simulink model "Autopilot_q_running1"  (R2021a)
settings: Solver=ode4  StartTime=0.0  StopTime=168  FixedStep=0.01  RelTol=1e-3
undefined symbols (not defined in the file or in its folder): Aero_cofficients, Earth, Plane_state_store, Structural_data, Thrust_data_store, WGS84
libraries: pid_lib x12, aerolibactuator x5, aerolibfltsims x2, aerolibanim x1, simulink x1, aerolibtransform2 x1, shared6dof x1, sim3dlib x1, uavsim3dlib x1
(part 2 of 3)

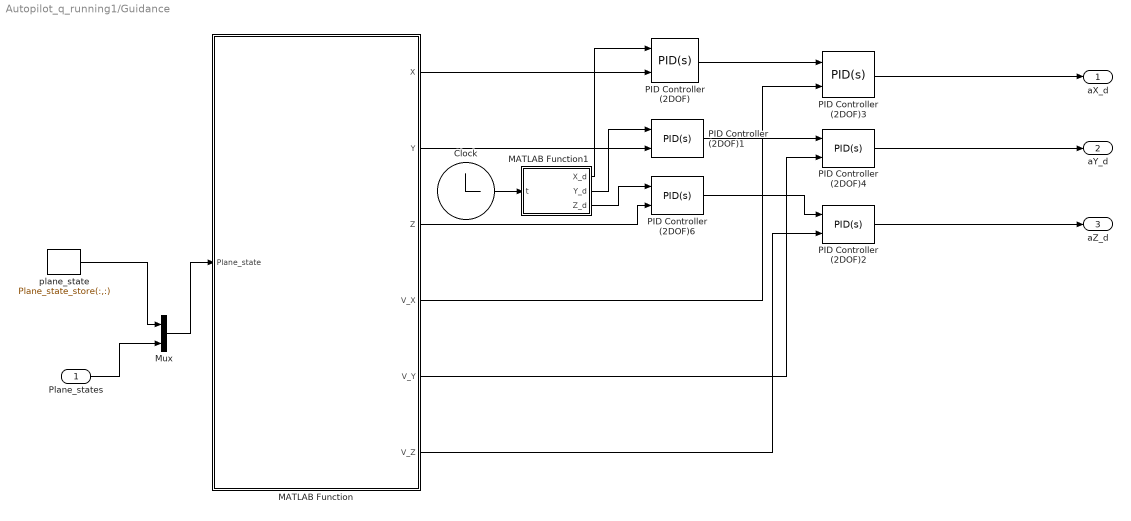
== system Autopilot_q_running1/Guidance ==
  Plane_states : Inport
  Clock : Clock
      settings: Decimation=200
  MATLAB Function : MATLAB Function  TreatAsAtomicUnit=on
  MATLAB Function1 : MATLAB Function  TreatAsAtomicUnit=on
  Mux : Mux  Inputs=2
  PID Controller (2DOF) : pid_lib/PID Controller (2DOF)  Controller=PID  Form=Parallel  TimeDomain=Continuous-time  UseExternalTs=off  SampleTime=-1  IntegratorMethod=Forward Euler  FilterMethod=Forward Euler  ControllerParametersSource=internal  P=0.4  I=0  D=0  UseFilter=on  N=100  b=1  c=1  TunerSelectOption=Transfer Function Based (PID Tuner App)  InitialConditionSource=internal  InitialConditionForIntegrator=0  InitialConditionForFilter=0  DifferentiatorICPrevScaledInput=0  ExternalReset=none  TrackingMode=off  Kt=1  LimitOutput=off  SatLimitsSource=internal  UpperSaturationLimit=inf  LowerSaturationLimit=-inf  LinearizeAsGain=on  AntiWindupMode=none  Kb=1  POutMin=[]  POutMax=[]  IOutMin=[]  IOutMax=[]  DOutMin=[]  DOutMax=[]  NOutMin=[]  NOutMax=[]  bOutMin=[]  bOutMax=[]  cOutMin=[]  cOutMax=[]  SumOutMin=[]  SumOutMax=[]  SaturationOutMin=[]  SaturationOutMax=[]  PParamMin=[]  PParamMax=[]  IParamMin=[]  IParamMax=[]  DParamMin=[]  DParamMax=[]  NParamMin=[]  NParamMax=[]  bParamMin=[]  bParamMax=[]  cParamMin=[]  cParamMax=[]  KbParamMin=[]  KbParamMax=[]  KtParamMin=[]  KtParamMax=[]  KbOutMin=[]  KbOutMax=[]  KtOutMin=[]  KtOutMax=[]  IntegratorOutMin=[]  IntegratorOutMax=[]  FilterOutMin=[]  FilterOutMax=[]  SumI1OutMin=[]  SumI1OutMax=[]  SumI2OutMin=[]  SumI2OutMax=[]  SumI3OutMin=[]  SumI3OutMax=[]  SumI4OutMin=[]  SumI4OutMax=[]  SumDOutMin=[]  SumDOutMax=[]  Sum1OutMin=[]  Sum1OutMax=[]  Sum2OutMin=[]  Sum2OutMax=[]  Sum3OutMin=[]  Sum3OutMax=[]  DifferentiatorOutMin=[]  DifferentiatorOutMax=[]  FilterDiffOutCoefMin=[]  FilterDiffOutCoefMax=[]  ReciprocalOutMin=[]  ReciprocalOutMax=[]  SumDenOutMin=[]  SumDenOutMax=[]  SumNumOutMin=[]  SumNumOutMax=[]  DivideOutMin=[]  DivideOutMax=[]  UdiffTsProdOutMin=[]  UdiffTsProdOutMax=[]  NTsProdOutMin=[]  NTsProdOutMax=[]  UintegralTsProdOutMin=[]  UintegralTsProdOutMax=[]  UngainTsProdOutMin=[]  UngainTsProdOutMax=[]  IntegratorContinuousStateAttributes=''  IntegratorStateMustResolveToSignalObject=off  IntegratorRTWStateStorageClass=Auto  FilterContinuousStateAttributes=''  FilterStateMustResolveToSignalObject=off  FilterRTWStateStorageClass=Auto  ParallelPVariant=InternalParameters  IdealPVariant=Disabled  IVariant=InternalParameters  DVariant=InternalParameters  bVariant=InternalParameters  cVariant=InternalParameters  IntegratorVariant=Continuous  SatVariant=Disabled  AWVariant=Passthrough  PCopyVariant=Disabled  TRVariant=Disabled  FdbkBlocksVariant=Forward  IdealPFdbkVariant=Disabled  SatFdbkVariant=Disabled  DerivativeFilterVariant=ContFilter  NVariant=InternalParameters  NCopyVariant=Disabled  FilterICVariant=InternalICsFilter  IntegratorICVariant=InternalICs  ExternalResetVariant=Disabled  TRSumVariant=Passthrough  SumFdbkVariant=Disabled  SumVariant=Sum_PID  TsampFilterVariant=InternalTs  TsampNgainVariant=Passthrough  TsampIntegralVariant=Passthrough  ExternalSaturationOutDataTypeStr=Inherit: Same as second input
      settings: SourceProductBaseCode=SL
  PID Controller (2DOF)1 : pid_lib/PID Controller (2DOF)  Controller=PID  Form=Parallel  TimeDomain=Continuous-time  UseExternalTs=off  SampleTime=-1  IntegratorMethod=Forward Euler  FilterMethod=Forward Euler  ControllerParametersSource=internal  P=0.4  I=0  D=0  UseFilter=on  N=100  b=1  c=1  TunerSelectOption=Transfer Function Based (PID Tuner App)  InitialConditionSource=internal  InitialConditionForIntegrator=0  InitialConditionForFilter=0  DifferentiatorICPrevScaledInput=0  ExternalReset=none  TrackingMode=off  Kt=1  LimitOutput=off  SatLimitsSource=internal  UpperSaturationLimit=inf  LowerSaturationLimit=-inf  LinearizeAsGain=on  AntiWindupMode=none  Kb=1  POutMin=[]  POutMax=[]  IOutMin=[]  IOutMax=[]  DOutMin=[]  DOutMax=[]  NOutMin=[]  NOutMax=[]  bOutMin=[]  bOutMax=[]  cOutMin=[]  cOutMax=[]  SumOutMin=[]  SumOutMax=[]  SaturationOutMin=[]  SaturationOutMax=[]  PParamMin=[]  PParamMax=[]  IParamMin=[]  IParamMax=[]  DParamMin=[]  DParamMax=[]  NParamMin=[]  NParamMax=[]  bParamMin=[]  bParamMax=[]  cParamMin=[]  cParamMax=[]  KbParamMin=[]  KbParamMax=[]  KtParamMin=[]  KtParamMax=[]  KbOutMin=[]  KbOutMax=[]  KtOutMin=[]  KtOutMax=[]  IntegratorOutMin=[]  IntegratorOutMax=[]  FilterOutMin=[]  FilterOutMax=[]  SumI1OutMin=[]  SumI1OutMax=[]  SumI2OutMin=[]  SumI2OutMax=[]  SumI3OutMin=[]  SumI3OutMax=[]  SumI4OutMin=[]  SumI4OutMax=[]  SumDOutMin=[]  SumDOutMax=[]  Sum1OutMin=[]  Sum1OutMax=[]  Sum2OutMin=[]  Sum2OutMax=[]  Sum3OutMin=[]  Sum3OutMax=[]  DifferentiatorOutMin=[]  DifferentiatorOutMax=[]  FilterDiffOutCoefMin=[]  FilterDiffOutCoefMax=[]  ReciprocalOutMin=[]  ReciprocalOutMax=[]  SumDenOutMin=[]  SumDenOutMax=[]  SumNumOutMin=[]  SumNumOutMax=[]  DivideOutMin=[]  DivideOutMax=[]  UdiffTsProdOutMin=[]  UdiffTsProdOutMax=[]  NTsProdOutMin=[]  NTsProdOutMax=[]  UintegralTsProdOutMin=[]  UintegralTsProdOutMax=[]  UngainTsProdOutMin=[]  UngainTsProdOutMax=[]  IntegratorContinuousStateAttributes=''  IntegratorStateMustResolveToSignalObject=off  IntegratorRTWStateStorageClass=Auto  FilterContinuousStateAttributes=''  FilterStateMustResolveToSignalObject=off  FilterRTWStateStorageClass=Auto  ParallelPVariant=InternalParameters  IdealPVariant=Disabled  IVariant=InternalParameters  DVariant=InternalParameters  bVariant=InternalParameters  cVariant=InternalParameters  IntegratorVariant=Continuous  SatVariant=Disabled  AWVariant=Passthrough  PCopyVariant=Disabled  TRVariant=Disabled  FdbkBlocksVariant=Forward  IdealPFdbkVariant=Disabled  SatFdbkVariant=Disabled  DerivativeFilterVariant=ContFilter  NVariant=InternalParameters  NCopyVariant=Disabled  FilterICVariant=InternalICsFilter  IntegratorICVariant=InternalICs  ExternalResetVariant=Disabled  TRSumVariant=Passthrough  SumFdbkVariant=Disabled  SumVariant=Sum_PID  TsampFilterVariant=InternalTs  TsampNgainVariant=Passthrough  TsampIntegralVariant=Passthrough  ExternalSaturationOutDataTypeStr=Inherit: Same as second input
      settings: SourceProductBaseCode=SL
  PID Controller (2DOF)2 : pid_lib/PID Controller (2DOF)  Controller=PID  Form=Parallel  TimeDomain=Continuous-time  UseExternalTs=off  SampleTime=-1  IntegratorMethod=Forward Euler  FilterMethod=Forward Euler  ControllerParametersSource=internal  P=1  I=0.0  D=0  UseFilter=on  N=100  b=1  c=1  TunerSelectOption=Transfer Function Based (PID Tuner App)  InitialConditionSource=internal  InitialConditionForIntegrator=0  InitialConditionForFilter=0  DifferentiatorICPrevScaledInput=0  ExternalReset=none  TrackingMode=off  Kt=1  LimitOutput=off  SatLimitsSource=internal  UpperSaturationLimit=inf  LowerSaturationLimit=-inf  LinearizeAsGain=on  AntiWindupMode=none  Kb=1  POutMin=[]  POutMax=[]  IOutMin=[]  IOutMax=[]  DOutMin=[]  DOutMax=[]  NOutMin=[]  NOutMax=[]  bOutMin=[]  bOutMax=[]  cOutMin=[]  cOutMax=[]  SumOutMin=[]  SumOutMax=[]  SaturationOutMin=[]  SaturationOutMax=[]  PParamMin=[]  PParamMax=[]  IParamMin=[]  IParamMax=[]  DParamMin=[]  DParamMax=[]  NParamMin=[]  NParamMax=[]  bParamMin=[]  bParamMax=[]  cParamMin=[]  cParamMax=[]  KbParamMin=[]  KbParamMax=[]  KtParamMin=[]  KtParamMax=[]  KbOutMin=[]  KbOutMax=[]  KtOutMin=[]  KtOutMax=[]  IntegratorOutMin=[]  IntegratorOutMax=[]  FilterOutMin=[]  FilterOutMax=[]  SumI1OutMin=[]  SumI1OutMax=[]  SumI2OutMin=[]  SumI2OutMax=[]  SumI3OutMin=[]  SumI3OutMax=[]  SumI4OutMin=[]  SumI4OutMax=[]  SumDOutMin=[]  SumDOutMax=[]  Sum1OutMin=[]  Sum1OutMax=[]  Sum2OutMin=[]  Sum2OutMax=[]  Sum3OutMin=[]  Sum3OutMax=[]  DifferentiatorOutMin=[]  DifferentiatorOutMax=[]  FilterDiffOutCoefMin=[]  FilterDiffOutCoefMax=[]  ReciprocalOutMin=[]  ReciprocalOutMax=[]  SumDenOutMin=[]  SumDenOutMax=[]  SumNumOutMin=[]  SumNumOutMax=[]  DivideOutMin=[]  DivideOutMax=[]  UdiffTsProdOutMin=[]  UdiffTsProdOutMax=[]  NTsProdOutMin=[]  NTsProdOutMax=[]  UintegralTsProdOutMin=[]  UintegralTsProdOutMax=[]  UngainTsProdOutMin=[]  UngainTsProdOutMax=[]  IntegratorContinuousStateAttributes=''  IntegratorStateMustResolveToSignalObject=off  IntegratorRTWStateStorageClass=Auto  FilterContinuousStateAttributes=''  FilterStateMustResolveToSignalObject=off  FilterRTWStateStorageClass=Auto  ParallelPVariant=InternalParameters  IdealPVariant=Disabled  IVariant=InternalParameters  DVariant=InternalParameters  bVariant=InternalParameters  cVariant=InternalParameters  IntegratorVariant=Continuous  SatVariant=Disabled  AWVariant=Passthrough  PCopyVariant=Disabled  TRVariant=Disabled  FdbkBlocksVariant=Forward  IdealPFdbkVariant=Disabled  SatFdbkVariant=Disabled  DerivativeFilterVariant=ContFilter  NVariant=InternalParameters  NCopyVariant=Disabled  FilterICVariant=InternalICsFilter  IntegratorICVariant=InternalICs  ExternalResetVariant=Disabled  TRSumVariant=Passthrough  SumFdbkVariant=Disabled  SumVariant=Sum_PID  TsampFilterVariant=InternalTs  TsampNgainVariant=Passthrough  TsampIntegralVariant=Passthrough  ExternalSaturationOutDataTypeStr=Inherit: Same as second input
      settings: SourceProductBaseCode=SL
  PID Controller (2DOF)3 : pid_lib/PID Controller (2DOF)  Controller=PID  Form=Parallel  TimeDomain=Continuous-time  UseExternalTs=off  SampleTime=-1  IntegratorMethod=Forward Euler  FilterMethod=Forward Euler  ControllerParametersSource=internal  P=1  I=0.0  D=0  UseFilter=on  N=100  b=1  c=1  TunerSelectOption=Transfer Function Based (PID Tuner App)  InitialConditionSource=internal  InitialConditionForIntegrator=0  InitialConditionForFilter=0  DifferentiatorICPrevScaledInput=0  ExternalReset=none  TrackingMode=off  Kt=1  LimitOutput=off  SatLimitsSource=internal  UpperSaturationLimit=inf  LowerSaturationLimit=-inf  LinearizeAsGain=on  AntiWindupMode=none  Kb=1  POutMin=[]  POutMax=[]  IOutMin=[]  IOutMax=[]  DOutMin=[]  DOutMax=[]  NOutMin=[]  NOutMax=[]  bOutMin=[]  bOutMax=[]  cOutMin=[]  cOutMax=[]  SumOutMin=[]  SumOutMax=[]  SaturationOutMin=[]  SaturationOutMax=[]  PParamMin=[]  PParamMax=[]  IParamMin=[]  IParamMax=[]  DParamMin=[]  DParamMax=[]  NParamMin=[]  NParamMax=[]  bParamMin=[]  bParamMax=[]  cParamMin=[]  cParamMax=[]  KbParamMin=[]  KbParamMax=[]  KtParamMin=[]  KtParamMax=[]  KbOutMin=[]  KbOutMax=[]  KtOutMin=[]  KtOutMax=[]  IntegratorOutMin=[]  IntegratorOutMax=[]  FilterOutMin=[]  FilterOutMax=[]  SumI1OutMin=[]  SumI1OutMax=[]  SumI2OutMin=[]  SumI2OutMax=[]  SumI3OutMin=[]  SumI3OutMax=[]  SumI4OutMin=[]  SumI4OutMax=[]  SumDOutMin=[]  SumDOutMax=[]  Sum1OutMin=[]  Sum1OutMax=[]  Sum2OutMin=[]  Sum2OutMax=[]  Sum3OutMin=[]  Sum3OutMax=[]  DifferentiatorOutMin=[]  DifferentiatorOutMax=[]  FilterDiffOutCoefMin=[]  FilterDiffOutCoefMax=[]  ReciprocalOutMin=[]  ReciprocalOutMax=[]  SumDenOutMin=[]  SumDenOutMax=[]  SumNumOutMin=[]  SumNumOutMax=[]  DivideOutMin=[]  DivideOutMax=[]  UdiffTsProdOutMin=[]  UdiffTsProdOutMax=[]  NTsProdOutMin=[]  NTsProdOutMax=[]  UintegralTsProdOutMin=[]  UintegralTsProdOutMax=[]  UngainTsProdOutMin=[]  UngainTsProdOutMax=[]  IntegratorContinuousStateAttributes=''  IntegratorStateMustResolveToSignalObject=off  IntegratorRTWStateStorageClass=Auto  FilterContinuousStateAttributes=''  FilterStateMustResolveToSignalObject=off  FilterRTWStateStorageClass=Auto  ParallelPVariant=InternalParameters  IdealPVariant=Disabled  IVariant=InternalParameters  DVariant=InternalParameters  bVariant=InternalParameters  cVariant=InternalParameters  IntegratorVariant=Continuous  SatVariant=Disabled  AWVariant=Passthrough  PCopyVariant=Disabled  TRVariant=Disabled  FdbkBlocksVariant=Forward  IdealPFdbkVariant=Disabled  SatFdbkVariant=Disabled  DerivativeFilterVariant=ContFilter  NVariant=InternalParameters  NCopyVariant=Disabled  FilterICVariant=InternalICsFilter  IntegratorICVariant=InternalICs  ExternalResetVariant=Disabled  TRSumVariant=Passthrough  SumFdbkVariant=Disabled  SumVariant=Sum_PID  TsampFilterVariant=InternalTs  TsampNgainVariant=Passthrough  TsampIntegralVariant=Passthrough  ExternalSaturationOutDataTypeStr=Inherit: Same as second input
      settings: SourceProductBaseCode=SL
  PID Controller (2DOF)4 : pid_lib/PID Controller (2DOF)  Controller=PID  Form=Parallel  TimeDomain=Continuous-time  UseExternalTs=off  SampleTime=-1  IntegratorMethod=Forward Euler  FilterMethod=Forward Euler  ControllerParametersSource=internal  P=1  I=0  D=0  UseFilter=on  N=100  b=1  c=1  TunerSelectOption=Transfer Function Based (PID Tuner App)  InitialConditionSource=internal  InitialConditionForIntegrator=0  InitialConditionForFilter=0  DifferentiatorICPrevScaledInput=0  ExternalReset=none  TrackingMode=off  Kt=1  LimitOutput=off  SatLimitsSource=internal  UpperSaturationLimit=inf  LowerSaturationLimit=-inf  LinearizeAsGain=on  AntiWindupMode=none  Kb=1  POutMin=[]  POutMax=[]  IOutMin=[]  IOutMax=[]  DOutMin=[]  DOutMax=[]  NOutMin=[]  NOutMax=[]  bOutMin=[]  bOutMax=[]  cOutMin=[]  cOutMax=[]  SumOutMin=[]  SumOutMax=[]  SaturationOutMin=[]  SaturationOutMax=[]  PParamMin=[]  PParamMax=[]  IParamMin=[]  IParamMax=[]  DParamMin=[]  DParamMax=[]  NParamMin=[]  NParamMax=[]  bParamMin=[]  bParamMax=[]  cParamMin=[]  cParamMax=[]  KbParamMin=[]  KbParamMax=[]  KtParamMin=[]  KtParamMax=[]  KbOutMin=[]  KbOutMax=[]  KtOutMin=[]  KtOutMax=[]  IntegratorOutMin=[]  IntegratorOutMax=[]  FilterOutMin=[]  FilterOutMax=[]  SumI1OutMin=[]  SumI1OutMax=[]  SumI2OutMin=[]  SumI2OutMax=[]  SumI3OutMin=[]  SumI3OutMax=[]  SumI4OutMin=[]  SumI4OutMax=[]  SumDOutMin=[]  SumDOutMax=[]  Sum1OutMin=[]  Sum1OutMax=[]  Sum2OutMin=[]  Sum2OutMax=[]  Sum3OutMin=[]  Sum3OutMax=[]  DifferentiatorOutMin=[]  DifferentiatorOutMax=[]  FilterDiffOutCoefMin=[]  FilterDiffOutCoefMax=[]  ReciprocalOutMin=[]  ReciprocalOutMax=[]  SumDenOutMin=[]  SumDenOutMax=[]  SumNumOutMin=[]  SumNumOutMax=[]  DivideOutMin=[]  DivideOutMax=[]  UdiffTsProdOutMin=[]  UdiffTsProdOutMax=[]  NTsProdOutMin=[]  NTsProdOutMax=[]  UintegralTsProdOutMin=[]  UintegralTsProdOutMax=[]  UngainTsProdOutMin=[]  UngainTsProdOutMax=[]  IntegratorContinuousStateAttributes=''  IntegratorStateMustResolveToSignalObject=off  IntegratorRTWStateStorageClass=Auto  FilterContinuousStateAttributes=''  FilterStateMustResolveToSignalObject=off  FilterRTWStateStorageClass=Auto  ParallelPVariant=InternalParameters  IdealPVariant=Disabled  IVariant=InternalParameters  DVariant=InternalParameters  bVariant=InternalParameters  cVariant=InternalParameters  IntegratorVariant=Continuous  SatVariant=Disabled  AWVariant=Passthrough  PCopyVariant=Disabled  TRVariant=Disabled  FdbkBlocksVariant=Forward  IdealPFdbkVariant=Disabled  SatFdbkVariant=Disabled  DerivativeFilterVariant=ContFilter  NVariant=InternalParameters  NCopyVariant=Disabled  FilterICVariant=InternalICsFilter  IntegratorICVariant=InternalICs  ExternalResetVariant=Disabled  TRSumVariant=Passthrough  SumFdbkVariant=Disabled  SumVariant=Sum_PID  TsampFilterVariant=InternalTs  TsampNgainVariant=Passthrough  TsampIntegralVariant=Passthrough  ExternalSaturationOutDataTypeStr=Inherit: Same as second input
      settings: SourceProductBaseCode=SL
  PID Controller (2DOF)6 : pid_lib/PID Controller (2DOF)  Controller=PID  Form=Parallel  TimeDomain=Continuous-time  UseExternalTs=off  SampleTime=-1  IntegratorMethod=Forward Euler  FilterMethod=Forward Euler  ControllerParametersSource=internal  P=.3  I=0.01  D=0  UseFilter=on  N=100  b=1  c=1  TunerSelectOption=Transfer Function Based (PID Tuner App)  InitialConditionSource=internal  InitialConditionForIntegrator=0  InitialConditionForFilter=0  DifferentiatorICPrevScaledInput=0  ExternalReset=none  TrackingMode=off  Kt=1  LimitOutput=off  SatLimitsSource=internal  UpperSaturationLimit=inf  LowerSaturationLimit=-inf  LinearizeAsGain=on  AntiWindupMode=none  Kb=1  POutMin=[]  POutMax=[]  IOutMin=[]  IOutMax=[]  DOutMin=[]  DOutMax=[]  NOutMin=[]  NOutMax=[]  bOutMin=[]  bOutMax=[]  cOutMin=[]  cOutMax=[]  SumOutMin=[]  SumOutMax=[]  SaturationOutMin=[]  SaturationOutMax=[]  PParamMin=[]  PParamMax=[]  IParamMin=[]  IParamMax=[]  DParamMin=[]  DParamMax=[]  NParamMin=[]  NParamMax=[]  bParamMin=[]  bParamMax=[]  cParamMin=[]  cParamMax=[]  KbParamMin=[]  KbParamMax=[]  KtParamMin=[]  KtParamMax=[]  KbOutMin=[]  KbOutMax=[]  KtOutMin=[]  KtOutMax=[]  IntegratorOutMin=[]  IntegratorOutMax=[]  FilterOutMin=[]  FilterOutMax=[]  SumI1OutMin=[]  SumI1OutMax=[]  SumI2OutMin=[]  SumI2OutMax=[]  SumI3OutMin=[]  SumI3OutMax=[]  SumI4OutMin=[]  SumI4OutMax=[]  SumDOutMin=[]  SumDOutMax=[]  Sum1OutMin=[]  Sum1OutMax=[]  Sum2OutMin=[]  Sum2OutMax=[]  Sum3OutMin=[]  Sum3OutMax=[]  DifferentiatorOutMin=[]  DifferentiatorOutMax=[]  FilterDiffOutCoefMin=[]  FilterDiffOutCoefMax=[]  ReciprocalOutMin=[]  ReciprocalOutMax=[]  SumDenOutMin=[]  SumDenOutMax=[]  SumNumOutMin=[]  SumNumOutMax=[]  DivideOutMin=[]  DivideOutMax=[]  UdiffTsProdOutMin=[]  UdiffTsProdOutMax=[]  NTsProdOutMin=[]  NTsProdOutMax=[]  UintegralTsProdOutMin=[]  UintegralTsProdOutMax=[]  UngainTsProdOutMin=[]  UngainTsProdOutMax=[]  IntegratorContinuousStateAttributes=''  IntegratorStateMustResolveToSignalObject=off  IntegratorRTWStateStorageClass=Auto  FilterContinuousStateAttributes=''  FilterStateMustResolveToSignalObject=off  FilterRTWStateStorageClass=Auto  ParallelPVariant=InternalParameters  IdealPVariant=Disabled  IVariant=InternalParameters  DVariant=InternalParameters  bVariant=InternalParameters  cVariant=InternalParameters  IntegratorVariant=Continuous  SatVariant=Disabled  AWVariant=Passthrough  PCopyVariant=Disabled  TRVariant=Disabled  FdbkBlocksVariant=Forward  IdealPFdbkVariant=Disabled  SatFdbkVariant=Disabled  DerivativeFilterVariant=ContFilter  NVariant=InternalParameters  NCopyVariant=Disabled  FilterICVariant=InternalICsFilter  IntegratorICVariant=InternalICs  ExternalResetVariant=Disabled  TRSumVariant=Passthrough  SumFdbkVariant=Disabled  SumVariant=Sum_PID  TsampFilterVariant=InternalTs  TsampNgainVariant=Passthrough  TsampIntegralVariant=Passthrough  ExternalSaturationOutDataTypeStr=Inherit: Same as second input
      settings: SourceProductBaseCode=SL
  plane_state : DataStoreRead  DataStoreName=Plane_state_store  DataStoreElements=Plane_state_store(:,:)  IndexOptions=Index vector (dialog)  Indices=1  OutputSizes=1
  aX_d : Outport  VectorParamsAs1DForOutWhenUnconnected=off
  aY_d : Outport  Port=2  VectorParamsAs1DForOutWhenUnconnected=off
  aZ_d : Outport  Port=3  VectorParamsAs1DForOutWhenUnconnected=off
  wires:
  MATLAB Function/1(X) -> PID Controller (2DOF)/2
  MATLAB Function/2(Y) -> PID Controller (2DOF)1/2
  MATLAB Function/3(Z) -> PID Controller (2DOF)6/2
  MATLAB Function/4(V_X) -> PID Controller (2DOF)3/2
  MATLAB Function/5(V_Y) -> PID Controller (2DOF)4/2
  MATLAB Function/6(V_Z) -> PID Controller (2DOF)2/2
  PID Controller (2DOF)/1 -> PID Controller (2DOF)3/1
  PID Controller (2DOF)1/1 -> PID Controller (2DOF)4/1
  PID Controller (2DOF)6/1 -> PID Controller (2DOF)2/1
  PID Controller (2DOF)3/1 -> aX_d/1
  PID Controller (2DOF)4/1 -> aY_d/1
  PID Controller (2DOF)2/1 -> aZ_d/1
  plane_state/1 -> Mux/1
  Plane_states/1 -> Mux/2
  Mux/1 -> MATLAB Function/1(Plane_state)
  MATLAB Function1/3(Z_d) -> PID Controller (2DOF)6/1
  MATLAB Function1/1(X_d) -> PID Controller (2DOF)/1
  MATLAB Function1/2(Y_d) -> PID Controller (2DOF)1/1
  Clock/1 -> MATLAB Function1/1(t)

== system Autopilot_q_running1/Plane_state_store ==
  Input : Inport
  Plane_state_data_write : DataStoreWrite  DataStoreName=Plane_state_store  DataStoreElements=Plane_state_store(:,:)  IndexOptions=Index vector (dialog)  Indices=1  OutputSizes=1
  wires:
  Input/1 -> Plane_state_data_write/1

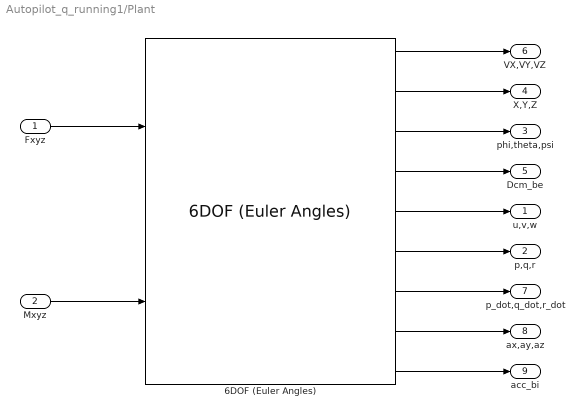
== system Autopilot_q_running1/Plant ==
  Fxyz : Inport
  Mxyz : Inport  Port=2
  6DOF (Euler Angles) : shared6dof/6DOF (Euler Angles)  units=Metric (MKS)  mtype=Fixed  rep=Euler Angles  xme_0=[0 0 0]  Vm_0=[0 0 0]  eul_0=[0 0 0/57.3]  pm_0=[0 0 0]  mass_0=25.0  mass_e=0.5  mass_f=2.0  inertia="[3.551, 0.1, 0; 0.1, 4.4221, 0; 0,  0, 7.7484]"  inertia_e=eye(3)  inertia_f=2*eye(3)  k_quat=1.0  vre_flag=on  abi_flag=on  aMode=0  xme_statename=''  Vm_statename=''  eul_statename=''  quat_statename=''  pm_statename=''  mass_statename=''
      settings: SourceProductBaseCode=AE,PW,DR,MT,UV,VE
  u,v,w : Outport  VectorParamsAs1DForOutWhenUnconnected=off
  p,q,r : Outport  Port=2  VectorParamsAs1DForOutWhenUnconnected=off
  phi,theta,psi : Outport  Port=3  VectorParamsAs1DForOutWhenUnconnected=off
  X,Y,Z : Outport  Port=4  VectorParamsAs1DForOutWhenUnconnected=off
  Dcm_be : Outport  Port=5  VectorParamsAs1DForOutWhenUnconnected=off
  VX,VY,VZ : Outport  Port=6  VectorParamsAs1DForOutWhenUnconnected=off
  p_dot,q_dot,r_dot : Outport  Port=7  VectorParamsAs1DForOutWhenUnconnected=off
  ax,ay,az : Outport  Port=8  VectorParamsAs1DForOutWhenUnconnected=off
  acc_bi : Outport  Port=9  VectorParamsAs1DForOutWhenUnconnected=off
  wires:
  Fxyz/1 -> 6DOF (Euler Angles)/1
  Mxyz/1 -> 6DOF (Euler Angles)/2
  6DOF (Euler Angles)/1 -> VX,VY,VZ/1
  6DOF (Euler Angles)/2 -> X,Y,Z/1
  6DOF (Euler Angles)/3 -> phi,theta,psi/1
  6DOF (Euler Angles)/4 -> Dcm_be/1
  6DOF (Euler Angles)/5 -> u,v,w/1
  6DOF (Euler Angles)/6 -> p,q,r/1
  6DOF (Euler Angles)/7 -> p_dot,q_dot,r_dot/1
  6DOF (Euler Angles)/8 -> ax,ay,az/1
  6DOF (Euler Angles)/9 -> acc_bi/1

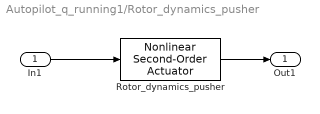
== system Autopilot_q_running1/Rotor_dynamics_pusher ==
  In1 : Inport
  Rotor_dynamics_pusher : aerolibactuator/Nonlinear Second-Order Actuator  wn_fin=200  z_fin=0.3  fin_max=25  fin_min=0  fin_maxrate=1000000  fin_act_0=0  fin_act_vel=0
      settings: SourceProductBaseCode=AE
  Out1 : Outport  VectorParamsAs1DForOutWhenUnconnected=off
  wires:
  In1/1 -> Rotor_dynamics_pusher/1
  Rotor_dynamics_pusher/1 -> Out1/1

== system Autopilot_q_running1/Rotor_dynamics_vtol_motors ==
  In1 : Inport
  Rotor_dynamics_vtol_motors : aerolibactuator/Nonlinear Second-Order Actuator  wn_fin=200  z_fin=0.5  fin_max=50000  fin_min=0  fin_maxrate=1000000  fin_act_0=0  fin_act_vel=0
      settings: SourceProductBaseCode=AE
  Out1 : Outport  VectorParamsAs1DForOutWhenUnconnected=off
  wires:
  In1/1 -> Rotor_dynamics_vtol_motors/1
  Rotor_dynamics_vtol_motors/1 -> Out1/1

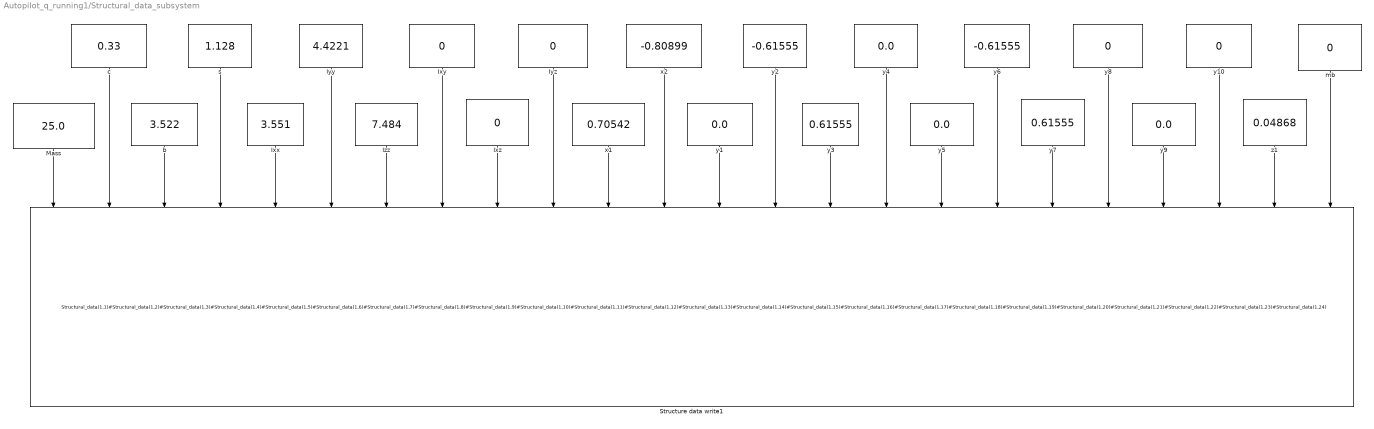
== system Autopilot_q_running1/Structural_data_subsystem ==
  Ixx : Constant  Value=3.551
  Ixy : Constant  Value=0
  Ixz : Constant  Value=0
  Iyy : Constant  Value=4.4221
  Iyz : Constant  Value=0
  Izz : Constant  Value=7.484
  Mass : Constant  Value=25.0
  Structure data write1 : DataStoreWrite  DataStoreName=Structural_data  DataStoreElements=Structural_data(1,1)#Structural_data(1,2)#Structural_data(1,3)#Structural_data(1,4)#Structural_data(1,5)#Structural_data(1,6)#Structural_data(1,7)#Structural_data(1,8)#Structural_data(1,9)#Structural_data(1,10)#Structural_data(1,11)#Structural_data(1,12)#Structural_data(1,13)#Structural_data(1,14)#Structural_data(1,15)#Structural_data(1,16)#Structural_data(1,17)#Structural_data(1,18)#Structural_data(1,19)#Structural_data(1,20)#Structural_data(1,21)#Structural_data(1,22)#Structural_data(1,23)#Structural_data(1,24)  IndexOptions=Index vector (dialog)  Indices=1  OutputSizes=1
  b : Constant  Value=3.522
  c : Constant  Value=0.33
  mb : Constant  Value=0
  s : Constant  Value=1.128
  x1 : Constant  Value=0.70542
  x2 : Constant  Value=-0.80899
  y{1,4..5,9} (4 alike) : Constant  Value=0.0
  y10 : Constant  Value=0
  y2 : Constant  Value=-0.61555
  y3 : Constant  Value=0.61555
  y6 : Constant  Value=-0.61555
  y7 : Constant  Value=0.61555
  y8 : Constant  Value=0
  z1 : Constant  Value=0.04868
  wires:
  Mass/1 -> Structure data write1/1
  c/1 -> Structure data write1/2
  b/1 -> Structure data write1/3
  Iyy/1 -> Structure data write1/6
  Ixx/1 -> Structure data write1/5
  s/1 -> Structure data write1/4
  Izz/1 -> Structure data write1/7
  Ixz/1 -> Structure data write1/9
  Ixy/1 -> Structure data write1/8
  Iyz/1 -> Structure data write1/10
  y8/1 -> Structure data write1/20
  y6/1 -> Structure data write1/18
  y7/1 -> Structure data write1/19
  y5/1 -> Structure data write1/17
  y2/1 -> Structure data write1/14
  y3/1 -> Structure data write1/15
  y4/1 -> Structure data write1/16
  y1/1 -> Structure data write1/13
  x2/1 -> Structure data write1/12
  x1/1 -> Structure data write1/11
  y9/1 -> Structure data write1/21
  z1/1 -> Structure data write1/23
  y10/1 -> Structure data write1/22
  mb/1 -> Structure data write1/24

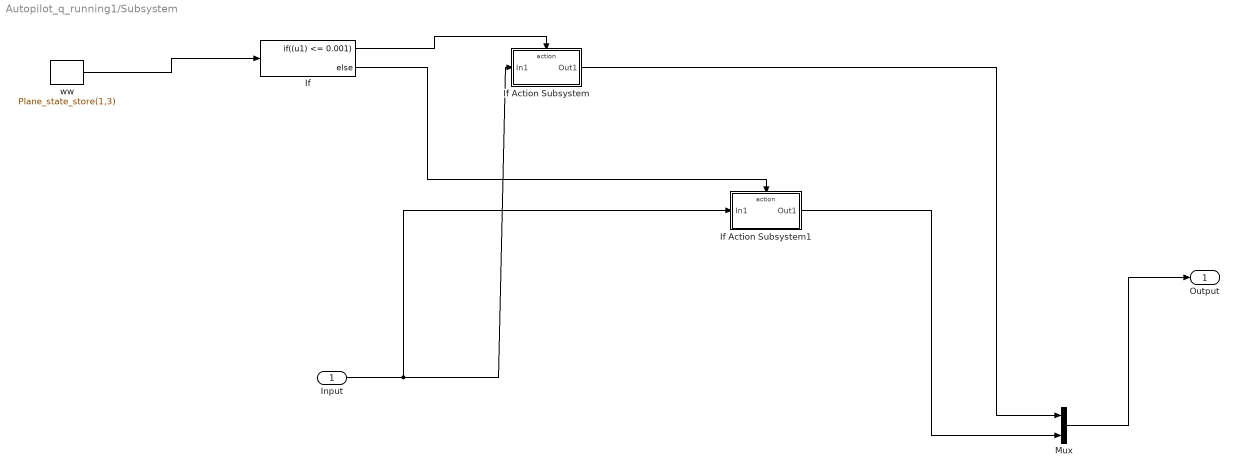
== system Autopilot_q_running1/Subsystem ==
  Input : Inport
  If : If  IfExpression=(u1) <= 0.001
  If Action Subsystem : Subsystem  TreatAsAtomicUnit=on
  If Action Subsystem1 : Subsystem  TreatAsAtomicUnit=on
  Mux : Mux  Inputs=2
  ww : DataStoreRead  DataStoreName=Plane_state_store  DataStoreElements=Plane_state_store(1,3)  IndexOptions=Index vector (dialog)  Indices=1  OutputSizes=1
  Output : Outport  VectorParamsAs1DForOutWhenUnconnected=off
  wires:
  ww/1 -> If/1
  If/1 -> If Action Subsystem/Action
  Input/1 -> If Action Subsystem1/1(In1), If Action Subsystem/1(In1)
  If/2 -> If Action Subsystem1/Action
  If Action Subsystem1/1(Out1) -> Mux/2
  If Action Subsystem/1(Out1) -> Mux/1
  Mux/1 -> Output/1

== system Autopilot_q_running1/Thrust_delta_store ==
  Input : Inport
  Thrust_data_store : DataStoreWrite  DataStoreName=Thrust_data_store  DataStoreElements=Thrust_data_store(:,:)  IndexOptions=Index vector (dialog)  Indices=1  OutputSizes=1
  wires:
  Input/1 -> Thrust_data_store/1

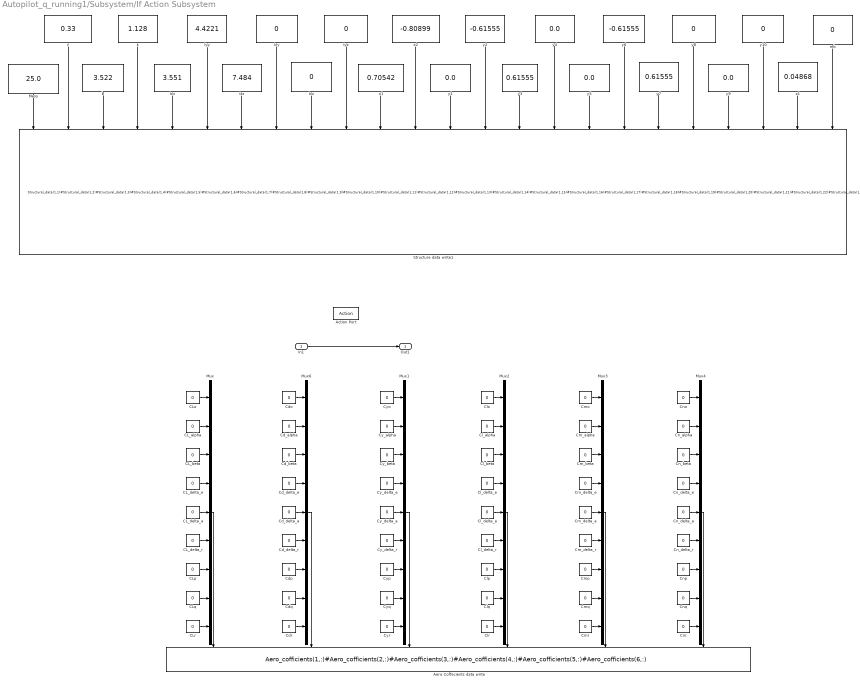
== system Autopilot_q_running1/Subsystem/If Action Subsystem ==
  In1 : Inport
  Action Port : ActionPort  ActionPortLabel=if((u1) <= 0.001)
  Aero Coffecients data write : DataStoreWrite  DataStoreName=Aero_cofficients  DataStoreElements=Aero_cofficients(1,:)#Aero_cofficients(2,:)#Aero_cofficients(3,:)#Aero_cofficients(4,:)#Aero_cofficients(5,:)#Aero_cofficients(6,:)  IndexOptions=Index vector (dialog)  Indices=1  OutputSizes=1
  CL_alpha : Constant  Value=0
  CL_beta : Constant  Value=0
  CL_delta_a : Constant  Value=0
  CL_delta_e : Constant  Value=0
  CL_delta_r : Constant  Value=0
  CLo : Constant  Value=0
  CLp : Constant  Value=0
  CLq : Constant  Value=0
  CLr : Constant  Value=0
  Cd_alpha : Constant  Value=0
  Cd_beta : Constant  Value=0
  Cd_delta_a : Constant  Value=0
  Cd_delta_e : Constant  Value=0
  Cd_delta_r : Constant  Value=0
  Cdo : Constant  Value=0
  Cdp : Constant  Value=0
  Cdq : Constant  Value=0
  Cdr : Constant  Value=0
  Cl_alpha : Constant  Value=0
  Cl_beta : Constant  Value=0
  Cl_delta_a : Constant  Value=0
  Cl_delta_e : Constant  Value=0
  Cl_delta_r : Constant  Value=0
  Clo : Constant  Value=0
  Clp : Constant  Value=0
  Clq : Constant  Value=0
  Clr : Constant  Value=0
  Cm_alpha : Constant  Value=0
  Cm_beta : Constant  Value=0
  Cm_delta_a : Constant  Value=0
  Cm_delta_e : Constant  Value=0
  Cm_delta_r : Constant  Value=0
  Cmo : Constant  Value=0
  Cmp : Constant  Value=0
  Cmq : Constant  Value=0
  Cmr : Constant  Value=0
  Cn_alpha : Constant  Value=0
  Cn_beta : Constant  Value=0
  Cn_delta_a : Constant  Value=0
  Cn_delta_e : Constant  Value=0
  Cn_delta_r : Constant  Value=0
  Cno : Constant  Value=0
  Cnp : Constant  Value=0
  Cnq : Constant  Value=0
  Cnr : Constant  Value=0
  Cy_alpha : Constant  Value=0
  Cy_beta : Constant  Value=0
  Cy_delta_a : Constant  Value=0
  Cy_delta_e : Constant  Value=0
  Cy_delta_r : Constant  Value=0
  Cyo : Constant  Value=0
  Cyp : Constant  Value=0
  Cyq : Constant  Value=0
  Cyr : Constant  Value=0
  Ixx : Constant  Value=3.551
  Ixy : Constant  Value=0
  Ixz : Constant  Value=0
  Iyy : Constant  Value=4.4221
  Iyz : Constant  Value=0
  Izz : Constant  Value=7.484
  Mass : Constant  Value=25.0
  Mux{,1..4,6} (6 alike) : Mux  Inputs=9
  Structure data write1 : DataStoreWrite  DataStoreName=Structural_data  DataStoreElements=Structural_data(1,1)#Structural_data(1,2)#Structural_data(1,3)#Structural_data(1,4)#Structural_data(1,5)#Structural_data(1,6)#Structural_data(1,7)#Structural_data(1,8)#Structural_data(1,9)#Structural_data(1,10)#Structural_data(1,11)#Structural_data(1,12)#Structural_data(1,13)#Structural_data(1,14)#Structural_data(1,15)#Structural_data(1,16)#Structural_data(1,17)#Structural_data(1,18)#Structural_data(1,19)#Structural_data(1,20)#Structural_data(1,21)#Structural_data(1,22)#Structural_data(1,23)#Structural_data(1,24)  IndexOptions=Index vector (dialog)  Indices=1  OutputSizes=1
  b : Constant  Value=3.522
  c : Constant  Value=0.33
  mb : Constant  Value=0
  s : Constant  Value=1.128
  x1 : Constant  Value=0.70542
  x2 : Constant  Value=-0.80899
  y{1,4..5,9} (4 alike) : Constant  Value=0.0
  y10 : Constant  Value=0
  y2 : Constant  Value=-0.61555
  y3 : Constant  Value=0.61555
  y6 : Constant  Value=-0.61555
  y7 : Constant  Value=0.61555
  y8 : Constant  Value=0
  z1 : Constant  Value=0.04868
  Out1 : Outport  VectorParamsAs1DForOutWhenUnconnected=off
  wires:
  In1/1 -> Out1/1
  Cn_delta_a/1 -> Mux4/5
  Cn_alpha/1 -> Mux4/2
  Mux3/1 -> Aero Coffecients data write/5
  Mux2/1 -> Aero Coffecients data write/4
  Cyo/1 -> Mux1/1
  Cn_beta/1 -> Mux4/3
  Cno/1 -> Mux4/1
  CLr/1 -> Mux/9
  Cnp/1 -> Mux4/7
  Cn_delta_r/1 -> Mux4/6
  Cm_delta_a/1 -> Mux3/5
  Cnq/1 -> Mux4/8
  Clp/1 -> Mux2/7
  Clo/1 -> Mux2/1
  Cm_alpha/1 -> Mux3/2
  Mux4/1 -> Aero Coffecients data write/6
  Cmo/1 -> Mux3/1
  Cnr/1 -> Mux4/9
  Cmq/1 -> Mux3/8
  Cl_delta_a/1 -> Mux2/5
  Cm_delta_r/1 -> Mux3/6
  CLq/1 -> Mux/8
  CL_delta_e/1 -> Mux/4
  Cmp/1 -> Mux3/7
  Cyr/1 -> Mux1/9
  Cl_delta_r/1 -> Mux2/6
  Mux1/1 -> Aero Coffecients data write/3
  Clq/1 -> Mux2/8
  CLo/1 -> Mux/1
  Cl_beta/1 -> Mux2/3
  Cy_alpha/1 -> Mux1/2
  Cy_delta_e/1 -> Mux1/4
  Mux/1 -> Aero Coffecients data write/1
  Cy_delta_r/1 -> Mux1/6
  Cm_delta_e/1 -> Mux3/4
  Cy_delta_a/1 -> Mux1/5
  CL_alpha/1 -> Mux/2
  Cd_alpha/1 -> Mux6/2
  Cm_beta/1 -> Mux3/3
  Cd_beta/1 -> Mux6/3
  Cyp/1 -> Mux1/7
  Cdp/1 -> Mux6/7
  Cd_delta_e/1 -> Mux6/4
  Mux6/1 -> Aero Coffecients data write/2
  Cd_delta_r/1 -> Mux6/6
  Cy_beta/1 -> Mux1/3
  Cyq/1 -> Mux1/8
  CL_delta_r/1 -> Mux/6
  Cd_delta_a/1 -> Mux6/5
  Cn_delta_e/1 -> Mux4/4
  Cdr/1 -> Mux6/9
  Cdq/1 -> Mux6/8
  Cl_alpha/1 -> Mux2/2
  Clr/1 -> Mux2/9
  CLp/1 -> Mux/7
  Cmr/1 -> Mux3/9
  Cl_delta_e/1 -> Mux2/4
  CL_delta_a/1 -> Mux/5
  CL_beta/1 -> Mux/3
  Cdo/1 -> Mux6/1
  y7/1 -> Structure data write1/19
  mb/1 -> Structure data write1/24
  Izz/1 -> Structure data write1/7
  y3/1 -> Structure data write1/15
  s/1 -> Structure data write1/4
  Ixy/1 -> Structure data write1/8
  Iyz/1 -> Structure data write1/10
  y8/1 -> Structure data write1/20
  y2/1 -> Structure data write1/14
  y4/1 -> Structure data write1/16
  x1/1 -> Structure data write1/11
  y9/1 -> Structure data write1/21
  y1/1 -> Structure data write1/13
  y6/1 -> Structure data write1/18
  y10/1 -> Structure data write1/22
  Ixx/1 -> Structure data write1/5
  Ixz/1 -> Structure data write1/9
  Mass/1 -> Structure data write1/1
  z1/1 -> Structure data write1/23
  b/1 -> Structure data write1/3
  y5/1 -> Structure data write1/17
  x2/1 -> Structure data write1/12
  c/1 -> Structure data write1/2
  Iyy/1 -> Structure data write1/6

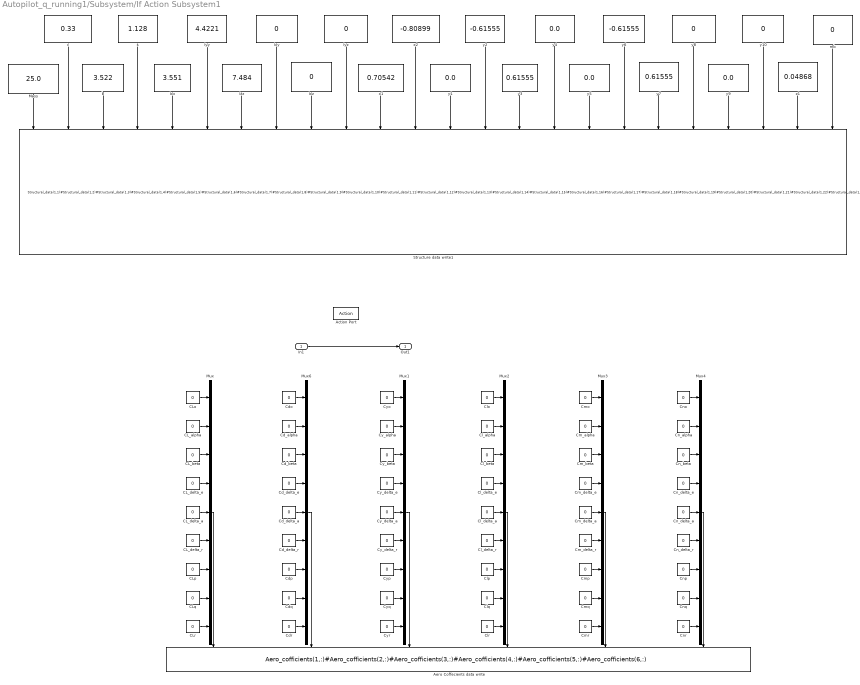
== system Autopilot_q_running1/Subsystem/If Action Subsystem1 ==
  In1 : Inport
  Action Port : ActionPort  ActionPortLabel=else
  Aero Coffecients data write : DataStoreWrite  DataStoreName=Aero_cofficients  DataStoreElements=Aero_cofficients(1,:)#Aero_cofficients(2,:)#Aero_cofficients(3,:)#Aero_cofficients(4,:)#Aero_cofficients(5,:)#Aero_cofficients(6,:)  IndexOptions=Index vector (dialog)  Indices=1  OutputSizes=1
  CL_alpha : Constant  Value=0
  CL_beta : Constant  Value=0
  CL_delta_a : Constant  Value=0
  CL_delta_e : Constant  Value=0
  CL_delta_r : Constant  Value=0
  CLo : Constant  Value=0
  CLp : Constant  Value=0
  CLq : Constant  Value=0
  CLr : Constant  Value=0
  Cd_alpha : Constant  Value=0
  Cd_beta : Constant  Value=0
  Cd_delta_a : Constant  Value=0
  Cd_delta_e : Constant  Value=0
  Cd_delta_r : Constant  Value=0
  Cdo : Constant  Value=0
  Cdp : Constant  Value=0
  Cdq : Constant  Value=0
  Cdr : Constant  Value=0
  Cl_alpha : Constant  Value=0
  Cl_beta : Constant  Value=0
  Cl_delta_a : Constant  Value=0
  Cl_delta_e : Constant  Value=0
  Cl_delta_r : Constant  Value=0
  Clo : Constant  Value=0
  Clp : Constant  Value=0
  Clq : Constant  Value=0
  Clr : Constant  Value=0
  Cm_alpha : Constant  Value=0
  Cm_beta : Constant  Value=0
  Cm_delta_a : Constant  Value=0
  Cm_delta_e : Constant  Value=0
  Cm_delta_r : Constant  Value=0
  Cmo : Constant  Value=0
  Cmp : Constant  Value=0
  Cmq : Constant  Value=0
  Cmr : Constant  Value=0
  Cn_alpha : Constant  Value=0
  Cn_beta : Constant  Value=0
  Cn_delta_a : Constant  Value=0
  Cn_delta_e : Constant  Value=0
  Cn_delta_r : Constant  Value=0
  Cno : Constant  Value=0
  Cnp : Constant  Value=0
  Cnq : Constant  Value=0
  Cnr : Constant  Value=0
  Cy_alpha : Constant  Value=0
  Cy_beta : Constant  Value=0
  Cy_delta_a : Constant  Value=0
  Cy_delta_e : Constant  Value=0
  Cy_delta_r : Constant  Value=0
  Cyo : Constant  Value=0
  Cyp : Constant  Value=0
  Cyq : Constant  Value=0
  Cyr : Constant  Value=0
  Ixx : Constant  Value=3.551
  Ixy : Constant  Value=0
  Ixz : Constant  Value=0
  Iyy : Constant  Value=4.4221
  Iyz : Constant  Value=0
  Izz : Constant  Value=7.484
  Mass : Constant  Value=25.0
  Mux{,1..4,6} (6 alike) : Mux  Inputs=9
  Structure data write1 : DataStoreWrite  DataStoreName=Structural_data  DataStoreElements=Structural_data(1,1)#Structural_data(1,2)#Structural_data(1,3)#Structural_data(1,4)#Structural_data(1,5)#Structural_data(1,6)#Structural_data(1,7)#Structural_data(1,8)#Structural_data(1,9)#Structural_data(1,10)#Structural_data(1,11)#Structural_data(1,12)#Structural_data(1,13)#Structural_data(1,14)#Structural_data(1,15)#Structural_data(1,16)#Structural_data(1,17)#Structural_data(1,18)#Structural_data(1,19)#Structural_data(1,20)#Structural_data(1,21)#Structural_data(1,22)#Structural_data(1,23)#Structural_data(1,24)  IndexOptions=Index vector (dialog)  Indices=1  OutputSizes=1
  b : Constant  Value=3.522
  c : Constant  Value=0.33
  mb : Constant  Value=0
  s : Constant  Value=1.128
  x1 : Constant  Value=0.70542
  x2 : Constant  Value=-0.80899
  y{1,4..5,9} (4 alike) : Constant  Value=0.0
  y10 : Constant  Value=0
  y2 : Constant  Value=-0.61555
  y3 : Constant  Value=0.61555
  y6 : Constant  Value=-0.61555
  y7 : Constant  Value=0.61555
  y8 : Constant  Value=0
  z1 : Constant  Value=0.04868
  Out1 : Outport  VectorParamsAs1DForOutWhenUnconnected=off
  wires:
  Iyy/1 -> Structure data write1/6
  c/1 -> Structure data write1/2
  x2/1 -> Structure data write1/12
  y5/1 -> Structure data write1/17
  b/1 -> Structure data write1/3
  z1/1 -> Structure data write1/23
  Mass/1 -> Structure data write1/1
  Ixz/1 -> Structure data write1/9
  Ixx/1 -> Structure data write1/5
  y10/1 -> Structure data write1/22
  y6/1 -> Structure data write1/18
  y1/1 -> Structure data write1/13
  y9/1 -> Structure data write1/21
  x1/1 -> Structure data write1/11
  y4/1 -> Structure data write1/16
  y2/1 -> Structure data write1/14
  y8/1 -> Structure data write1/20
  Iyz/1 -> Structure data write1/10
  Ixy/1 -> Structure data write1/8
  s/1 -> Structure data write1/4
  y3/1 -> Structure data write1/15
  Izz/1 -> Structure data write1/7
  mb/1 -> Structure data write1/24
  y7/1 -> Structure data write1/19
  Cdo/1 -> Mux6/1
  CL_beta/1 -> Mux/3
  CL_delta_a/1 -> Mux/5
  Cl_delta_e/1 -> Mux2/4
  Cmr/1 -> Mux3/9
  CLp/1 -> Mux/7
  Clr/1 -> Mux2/9
  Cl_alpha/1 -> Mux2/2
  Cdq/1 -> Mux6/8
  Cdr/1 -> Mux6/9
  Cn_delta_e/1 -> Mux4/4
  Cd_delta_a/1 -> Mux6/5
  CL_delta_r/1 -> Mux/6
  Cyq/1 -> Mux1/8
  Cy_beta/1 -> Mux1/3
  Cd_delta_r/1 -> Mux6/6
  Mux6/1 -> Aero Coffecients data write/2
  Cd_delta_e/1 -> Mux6/4
  Cdp/1 -> Mux6/7
  Cyp/1 -> Mux1/7
  Cd_beta/1 -> Mux6/3
  Cm_beta/1 -> Mux3/3
  Cd_alpha/1 -> Mux6/2
  CL_alpha/1 -> Mux/2
  Cy_delta_a/1 -> Mux1/5
  Cm_delta_e/1 -> Mux3/4
  Cy_delta_r/1 -> Mux1/6
  Mux/1 -> Aero Coffecients data write/1
  Cy_delta_e/1 -> Mux1/4
  Cy_alpha/1 -> Mux1/2
  Cl_beta/1 -> Mux2/3
  CLo/1 -> Mux/1
  Clq/1 -> Mux2/8
  Mux1/1 -> Aero Coffecients data write/3
  Cl_delta_r/1 -> Mux2/6
  Cyr/1 -> Mux1/9
  Cmp/1 -> Mux3/7
  CL_delta_e/1 -> Mux/4
  CLq/1 -> Mux/8
  Cm_delta_r/1 -> Mux3/6
  Cl_delta_a/1 -> Mux2/5
  Cmq/1 -> Mux3/8
  Cnr/1 -> Mux4/9
  Cmo/1 -> Mux3/1
  Mux4/1 -> Aero Coffecients data write/6
  Cm_alpha/1 -> Mux3/2
  Clo/1 -> Mux2/1
  Clp/1 -> Mux2/7
  Cnq/1 -> Mux4/8
  Cm_delta_a/1 -> Mux3/5
  Cn_delta_r/1 -> Mux4/6
  Cnp/1 -> Mux4/7
  CLr/1 -> Mux/9
  Cno/1 -> Mux4/1
  Cn_beta/1 -> Mux4/3
  Cyo/1 -> Mux1/1
  Mux2/1 -> Aero Coffecients data write/4
  Mux3/1 -> Aero Coffecients data write/5
  Cn_alpha/1 -> Mux4/2
  Cn_delta_a/1 -> Mux4/5
  In1/1 -> Out1/1

== matlab function Autopilot_q_running1/Guidance/MATLAB Function1 ==
  data: X_d output; Y_d output; t input; Z_d output
function [X_d,Y_d,Z_d] = fcn(t)
tf0=0;
tf1=30.0;
tf2=35.0;
tf3=132.0;
tf4=172.0;
tf5=190.0;
circle_mode=1;
cruise_mode=0;


Z_i_takeoff=0.0;
Z_f_takeoff=-50.0;
Z_i_landing=-50.0;
Z_f_landing=0.0;


Z_d=0.0;
X_d=0;
Y_d=0;

if t>=tf0 && t<tf1
X_d=0;
Y_d=0;
Z_d=Z_i_takeoff + 2*(Z_f_takeoff-Z_i_takeoff)*(t-tf0)/(tf1-tf0) +((Z_i_takeoff-Z_f_takeoff)*((t-tf0)^2)/((tf1-tf0)^2)) ;
end

if t>=tf1 && t<tf2
X_d=0;
Y_d=0;
Z_d=Z_f_takeoff;
end

if circle_mode==1

if t>=tf2 && t<tf3
        R_circ=25;
		Z_d = -50;%Z_i_circle;
		X_d = R_circ*sin((t-tf2)*((2*pi)/(tf3-tf2)));% + X_i_circle;
		Y_d = R_circ*cos((t-tf2)*((2*pi)/(tf3-tf2)))- R_circ;% + Y_i_circle - R_circ;
end

if t>=tf3 && t<=tf4
X_d=0;
Y_d=0;
Z_d=Z_i_landing + 2*(Z_f_landing-Z_i_landing)*(t-tf3)/(tf4-tf3) +((Z_i_landing-Z_f_landing)*((t-tf3)^2)/((tf4-tf3)^2)) ;
end


end


if cruise_mode==1
    
    
if t>=tf2 && t<tf3
X_d=10*(t-tf2);
Y_d=0.0;
Z_d=Z_f_takeoff;
    
end


if t>=tf3 && t<tf4
V_x_tf3 = 10;  
x_tf3 = 80;
X_d= (V_x_tf3/(2*(tf3-tf4)))*t^2 + (V_x_tf3*tf4/(tf4-tf3))*t  + x_tf3 - (V_x_tf3/(2*(tf3-tf4)))*tf3^2 - (V_x_tf3*tf4/(tf4-tf3))*tf3 ;
Y_d=0.0;
Z_d=Z_f_takeoff;
end

if t>=tf4 && t<=tf5
    V_x_tf3 = 10;  
    x_tf3 = 80;
    X_d=(V_x_tf3/(2*(tf3-tf4)))*tf4^2 + (V_x_tf3*tf4/(tf4-tf3))*tf4  + x_tf3 - (V_x_tf3/(2*(tf3-tf4)))*tf3^2 - (V_x_tf3*tf4/(tf4-tf3))*tf3 ;
    Y_d=0.0;
    Z_d=Z_i_landing + 2*(Z_f_landing-Z_i_landing)*(t-tf4)/(tf4-tf4) +((Z_i_landing-Z_f_landing)*((t-tf4)^2)/((tf5-tf4)^2)) ;
end
end


end

== matlab function Autopilot_q_running1/Autopilot Quad mode/MATLAB Function1 ==
  data: t input; TT input; mass input; a_y_d input; phi_d output
function phi_d  = fcn(t, TT, mass, a_y_d)
TT=sum(TT);
if (abs(TT)<1)
    TT=1;
end
while (abs(mass*a_y_d/TT)) >= 0.7 %% 45 deg max
    TT=TT+1;
end
phi_d=asin((mass/TT)*a_y_d);

end

== matlab function Autopilot_q_running1/Autopilot Quad mode/MATLAB Function2 ==
  data: angular_state input; phi_dot_d input; p_d output
function p_d  = fcn(angular_state,phi_dot_d)
p=angular_state(1);
q=angular_state(2);
r=angular_state(3);
phi=angular_state(4);
theta=angular_state(5);
psi=angular_state(6);
p_d= phi_dot_d - q*sin(phi)*tan(theta)-r*cos(phi)*tan(theta);

end

== matlab function Autopilot_q_running1/Autopilot Quad mode/MATLAB Function3 ==
  data: t input; TT input; mass input; a_x_d input; theta_d output
function theta_d  = fcn(t, TT, mass, a_x_d)
TT=sum(TT);
if (abs(TT)<1)
    TT=1;
end
while (abs(mass*a_x_d/TT)) >= 0.7 %% 45 deg max
    TT=TT+1;
end
theta_d=asin(-(mass/TT)*a_x_d);



end

== matlab function Autopilot_q_running1/Autopilot Quad mode/MATLAB Function4 ==
  data: angular_state input; theta_dot_d input; q_d output
function q_d  = fcn(angular_state,theta_dot_d)

p=angular_state(1);
q=angular_state(2);
r=angular_state(3);
phi=angular_state(4);
theta=angular_state(5);
psi=angular_state(6);

if (abs(phi)>(pi/2.5))
		
	q_d=(theta_dot_d +r*sin(phi));
		
else
		
	q_d=(theta_dot_d +r*sin(phi))/cos(phi);
end

end

== matlab function Autopilot_q_running1/Autopilot Quad mode/MATLAB Function5 ==
  data: t input; psi_d output; u input; v input
function psi_d  = fcn(t,u,v)
psi_d=0;

if t>=35 && t<60
psi_d= -(pi/50)*(t-35);
end


if t>=60 && t<85
    psi_d= -(pi/2) - (pi/50)*(t-60);
end

if t>=85 && t<110
    psi_d= (pi) - (pi/50)*(t-85);
end

if t>=110 && t<135
    psi_d= (pi/2) - (pi/50)*(t-110);
end
    




end

== matlab function Autopilot_q_running1/Autopilot Quad mode/MATLAB Function6 ==
  data: angular_state input; psi_dot_d input; r_d output
function r_d  = fcn(angular_state,psi_dot_d)

p=angular_state(1);
q=angular_state(2);
r=angular_state(3);
phi=angular_state(4);
theta=angular_state(5);
psi=angular_state(6);
if (abs(phi)>=((89.0)/57.3))
    phi=abs(phi)*89.0/(57.3*phi);
end
r_d = (psi_dot_d - q*sin(phi)*sec(theta))/(cos(phi)*sec(theta));
end

== matlab function Autopilot_q_running1/Autopilot Quad mode/MATLAB Function ==
  data: psi_d input; psi_error output; psi input
function psi_error = fcn(psi_d, psi)

psi_error=psi_d-psi;

if ( abs(psi_error) > pi )
    psi_error = -(psi_error/(abs(psi_error)))*abs((2*pi) - abs(psi_error));
end

end

== matlab function Autopilot_q_running1/Autopilot Quad mode/MATLAB Function7 ==
  data: Plane_state input; u1 input; u_dot_d output; v_dot_d output; w_dot_d output
function [u_dot_d,v_dot_d,w_dot_d] = fcn(Plane_state, u1)

phi=Plane_state(7);
theta=Plane_state(8);
psi=Plane_state(9);




R_v_v1=[cos(psi) sin(psi) 0; -sin(psi) cos(psi) 0; 0 0 1];
R_v1_v2=[cos(theta) 0 -sin(theta) ;0 1 0; sin(theta) 0 cos(theta)];
R_v2_b=[1 0 0;0 cos(phi) sin(phi) ;0 -sin(phi) cos(phi)];
R_v_b=R_v2_b*R_v1_v2*R_v_v1;

AA=zeros(3,1);

AA=R_v_b*u1';

u_dot_d=AA(1);
v_dot_d=AA(2);
w_dot_d=AA(3);

end

== matlab function Autopilot_q_running1/MATLAB Function ==
  data: u input; phi output; theta output; u1 input
function [phi,theta] = fcn(u, u1)
ax=u(4);%acc
ay=u(5);
az=u(6);

p=u(1);%gyro
q=u(2);
%r=u(3);
acc=5000;
gy=70;

theta = 0;
phi = 0;
phi_original=u1(1);
theta_original=u1(2);

dt=0.01;
 theta= theta + q*dt;
 phi= phi- p*dt;
 
    phiacc= atan(ax/ay);
    
    phi=phi*0.98+phiacc*0.02;
    
    thetaacc=atan(ay/ax);
    
    theta=theta*0.98+thetaacc*0.02;
    phi = phi_original - phi * 57.3;
    theta = theta_original - theta * 57.3;
end

== matlab function Autopilot_q_running1/Guidance/MATLAB Function ==
  data: Plane_state input; X output; Y output; Z output; V_X output; V_Y output; V_Z output
function [X,Y,Z,V_X,V_Y,V_Z] = fcn(Plane_state)

X=Plane_state(10);
Y=Plane_state(11);
Z=Plane_state(12);
V_X=Plane_state(13);
V_Y=Plane_state(14);
V_Z=Plane_state(15);

end

== matlab function Autopilot_q_running1/Forces and moments/Forces and moments ==
  data: Tzf1 input; Tzf2 input; Tzf3 input; Tzf4 input; Tzb5 input; Tzb6 input; Tzb7 input; Tzb8 input; Tx9 input; Tx10 input; delta_e input; delta_a input; delta_r input; fx output; fy output; fz output; l output; m output; n output; aero_data input; structure_data input; ideal_Plane_state input
function [fx,fy,fz,l,m,n] = fcn(Tzf1,Tzf2,Tzf3,Tzf4,Tzb5,Tzb6,Tzb7,Tzb8,Tx9,Tx10,delta_e,delta_a,delta_r, aero_data,structure_data , ideal_Plane_state)

mass=structure_data(1,1);c=structure_data(1,2);b=structure_data(1,3);s=structure_data(1,4);
Ix=structure_data(1,5);Iy=structure_data(1,6);Iz=structure_data(1,7);
Ixy=structure_data(1,8);Ixz=structure_data(1,9);Iyz=structure_data(1,10);
x1=structure_data(1,11);x2=structure_data(1,12);y1=structure_data(1,13);y2=structure_data(1,14);
y3=structure_data(1,15);y4=structure_data(1,16);y5=structure_data(1,17);y6=structure_data(1,18);
y7=structure_data(1,19);y8=structure_data(1,20);y9=structure_data(1,21);y10=structure_data(1,22);
z1=structure_data(1,23);mb=structure_data(1,24);

c0=Ix*Iz-Ixz^2; 
c1=Ixz*(Ix-Iy+Iz)/c0;    
c2=(Iz*(Iz-Iy)+Ixz^2)/c0;                                              
c3=Iz/c0;
c4=Ixz/c0;
c5=(Iz-Ix)/c0;
c6=Ixz/Iy;
c7=((Ix-Iy)*Ix + Ixz^2)/c0;
c8=Ix/c0;

CLo =aero_data(1,1); CL_alpha=aero_data(1,2);CL_beta=aero_data(1,3); CL_delta_e=aero_data(1,4); CL_delta_a=aero_data(1,5); CL_delta_r=aero_data(1,6); CL_p=aero_data(1,7);CL_q=aero_data(1,8);CL_r=aero_data(1,9);

Cdo =aero_data(1,1); Cd_alpha=aero_data(1,2);Cd_beta=aero_data(1,3); Cd_delta_e=aero_data(1,4); Cd_delta_a=aero_data(1,5); Cd_delta_r=aero_data(1,6); Cd_p=aero_data(1,7);Cd_q=aero_data(1,8);Cd_r=aero_data(1,9);

CYo =aero_data(1,1); CY_alpha=aero_data(1,2);CY_beta=aero_data(1,3); CY_delta_e=aero_data(1,4); CY_delta_a=aero_data(1,5); CY_delta_r=aero_data(1,6); CY_p=aero_data(1,7);CY_q=aero_data(1,8);CY_r=aero_data(1,9);

Clo =aero_data(1,1); Cl_alpha=aero_data(1,2);Cl_beta=aero_data(1,3); Cl_delta_e=aero_data(1,4); Cl_delta_a=aero_data(1,5); Cl_delta_r=aero_data(1,6); Cl_p=aero_data(1,7);Cl_q=aero_data(1,8);Cl_r=aero_data(1,9);

Cmo =aero_data(1,1); Cm_alpha=aero_data(1,2);Cm_beta=aero_data(1,3); Cm_delta_e=aero_data(1,4); Cm_delta_a=aero_data(1,5); Cm_delta_r=aero_data(1,6); Cm_p=aero_data(1,7);Cm_q=aero_data(1,8);Cm_r=aero_data(1,9);

Cno =aero_data(1,1); Cn_alpha=aero_data(1,2);Cn_beta=aero_data(1,3); Cn_delta_e=aero_data(1,4); Cn_delta_a=aero_data(1,5); Cn_delta_r=aero_data(1,6); Cn_p=aero_data(1,7);Cn_q=aero_data(1,8);Cn_r=aero_data(1,9);

Cd_brake=0.0;brake=0.0;g=9.81;
b1=0.0007488;
d1=0.00002828;
b1_inv=1.0/b1;

u=ideal_Plane_state(1);
v=ideal_Plane_state(2);
w=ideal_Plane_state(3);
p=ideal_Plane_state(4);
q=ideal_Plane_state(5);
r=ideal_Plane_state(6);
phi=ideal_Plane_state(7);
theta=ideal_Plane_state(8);
psi=ideal_Plane_state(9);
X=ideal_Plane_state(10);
Y=ideal_Plane_state(11);
Z=ideal_Plane_state(12);



rho=1.225;
Tzf=Tzf2+Tzf3;
Tzb=Tzb6+Tzb7; 


R_v_v1=[cos(psi) sin(psi) 0; -sin(psi) cos(psi) 0; 0 0 1];
R_v1_v2=[cos(theta) 0 -sin(theta) ;0 1 0; sin(theta) 0 cos(theta)];
R_v2_b=[1 0 0;0 cos(phi) sin(phi) ;0 -sin(phi) cos(phi)];
R_v_b=R_v2_b*R_v1_v2*R_v_v1;



V_v=R_v_b'*[ u;  v;  w];
V_X=V_v(1);
V_Y=V_v(2);
V_Z=V_v(3);
wn=0.0;
we=0.0;
wd=0.0;
ppp = R_v_b*[V_X-wn;V_Y-we;V_Z-wd];
u_r=ppp(1);
v_r=ppp(2);
w_r=ppp(3);

V=sqrt(u_r^2+v_r^2+w_r^2);



if (u_r^2+v_r^2+w_r^2)<=0.01 
    alpha=0;
else
    alpha=atan2( w_r, u_r);
end


if norm(u_r) < 10^-3  && norm(v_r) < 10^-3 && norm(w_r) < 10^-3
    beta=0;
else
    beta = asin(v_r/sqrt(u_r^2+v_r^2+w_r^2));
end



R_b_s=[cos(alpha) 0 sin(alpha) ;0 1 0; -sin(alpha) 0 cos(alpha)]; 
R_s_w=[cos(beta) sin(beta) 0; -sin(beta) cos(beta) 0; 0 0 1];
R_w_b=(R_b_s)'*(R_s_w)';




mg_b = R_v_b*[0 ;0; mass*g];
D=0.5*rho*V*V*s*(Cdo+Cd_alpha*abs(alpha)+Cd_delta_e*abs(delta_e)+ Cd_brake*abs(brake)) ;
D_b=R_w_b*[-D;0;0];

if V<0.1
    CL = CLo + CL_alpha*alpha + CL_delta_e*delta_e ;
else
    CL = CLo + CL_alpha*alpha + CL_delta_e*delta_e  + CL_q*q*c/(2*V) ;
end
L=0.5*rho*V*V*s*(CL);
L_b = R_w_b*[0;0;-L];
if abs(V)<0.1
    CY=CYo + CY_delta_r*delta_r + CY_beta*beta;
else
    CY=CYo + CY_delta_r*delta_r + CY_beta*beta + CY_r*r*b/(2*V);
end
FY=0.5*rho*V*V*s*(CY);

l_aero=0.5*rho*V^2*s*b*( Clo + Cl_delta_a*delta_a +Cl_delta_r*delta_r +Cl_beta*beta )+0.5*rho*V*s*b*(Cl_p*p*b/2+Cl_r*r*b/2);
m_aero=0.5*rho*V^2*s*c*( Cmo + Cm_alpha*alpha + Cm_delta_e*delta_e)+0.5*rho*V*s*c*Cm_q*q*c/2;
n_aero=0.5*rho*V^2*s*b*( Cno + Cn_delta_a*delta_a +Cn_delta_r*delta_r +Cn_beta*beta )+0.5*rho*V*s*b*(Cn_r*r*b/2+ Cn_p*p*b/2);

    
	l=l_aero - Tzf2*y2*cos(mb) - Tzf3*y3*cos(mb)   - Tzb6*y6*cos(mb) - Tzb7*y7*cos(mb);
	m=m_aero + Tzf*x1*cos(mb) + Tzb*x2*cos(mb) + Tx9*z1 + d1*Tzf2*b1_inv*sin(mb) - d1*Tzf3*b1_inv*sin(mb) - d1*Tzb6*b1_inv*sin(mb) + d1*Tzb7*b1_inv*sin(mb) ;
%	n=n_aero - Tx9_real*y9  - d1*Tzf2_real/b1 + d1*Tzf3_real/b1 + d1*Tzb6_real/b1 - d1*Tzb7_real/b1 ; //optimization
	n=n_aero - Tx9*y9 - Tx10*y10 + (Tzf2*x1*sin(mb) - Tzf3*x1*sin(mb) +  Tzb6*x2*sin(mb) - Tzb7*x2*sin(mb)) - d1*Tzf2*b1_inv*cos(mb) + d1*Tzf3*b1_inv*cos(mb)  + d1*Tzb6*b1_inv*cos(mb)  - d1*Tzb7*b1_inv*cos(mb)  ;



	fx = Tx9 + Tx10 + D_b(1)+ mg_b(1)+L_b(1);
	%%%%%%%%%%%%%%%%%%%%%%%%%%%%%%%%%%%%%%%%%%%%%%%%%%%%%%%%%%%%%%%%%%%%%%%%%%%
	fy = (Tzf2*sin(mb) - Tzf3*sin(mb) + Tzb6*sin(mb) - Tzb7*sin(mb)) + D_b(2) + mg_b(2) + FY + L_b(2);
	%%%%%%%%%%%%%%%%%%%%%%%%%%%%%%%%%%%%%%%%%%%%%%%%%%%%%%%%%%%%%%%%%%%%%%%%%%%
	fz = -Tzf*cos(mb) - Tzb*cos(mb) + mg_b(3)+D_b(3)+L_b(3);

    

end
